simulink model "Scope"  (R2024a)
settings: Solver=VariableStepAuto  StartTime=0.0  StopTime=inf  RelTol=1e-3
undefined symbols (not defined in the file or in its folder): HA
libraries: Visualization x1
settings Model: Creator=teruk  LastModifiedBy=djbranglab-ucsf

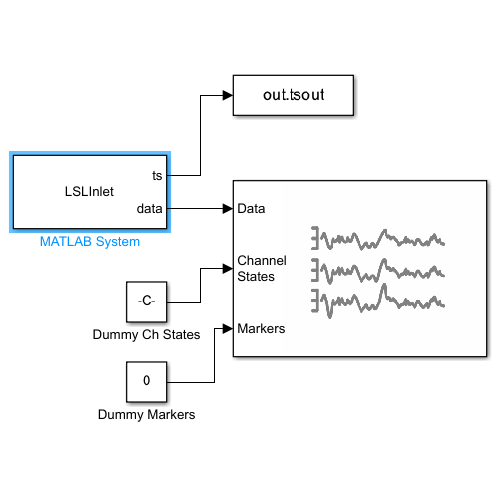
[thumbnail: Simulink's stored preview of the top-level diagram]
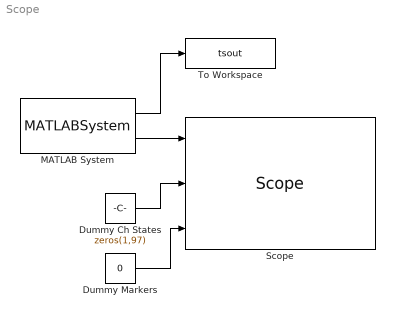
== system Scope ==
  Dummy Ch States : Constant  Value=zeros(1,97)
  Dummy Markers : Constant  Value=0
  MATLAB System : MATLABSystem  System=LSLInlet  StreamType=EEG  SourceID=HA-2016.03.01  NumChannels=97  Fs=4800  SimulateUsing=Interpreted execution
      mask Type: LSLInlet
      mask Display:
      | disp('LSLInlet');
      | port_label('output',1,'ts');
      | port_label('output',2,'data');
  Scope : Visualization/Scope
      settings: SourceProductName=Visualization
  To Workspace : ToWorkspace  VariableName=tsout  SampleTime=-1
  wires:
  Dummy Markers/1 -> Scope/3
  Dummy Ch States/1 -> Scope/2
  MATLAB System/2 -> Scope/1
  MATLAB System/1 -> To Workspace/1
